simulink model "prob1"  (R2020b)
settings: Solver=VariableStepAuto  StartTime=0.0  StopTime=10.0  RelTol=1e-3
undefined symbols (not defined in the file): M1
settings Model: Creator=nadee  LastModifiedBy=nadee

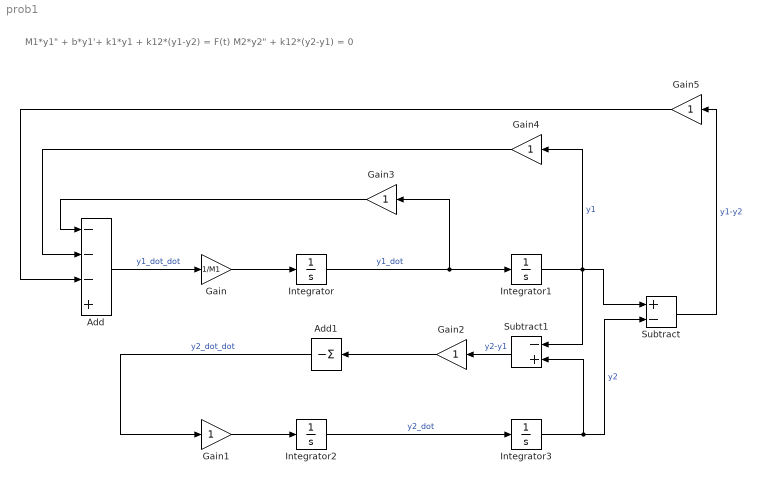
== system prob1 ==
  note: M1*y1" + b*y1'+ k1*y1 + k12*(y1-y2) = F(t)
      | M2*y2" + k12*(y2-y1) = 0
  Add : Sum  Inputs=---+
  Add1 : Sum  Inputs=-
  Gain : Gain  Gain=1/M1
  Gain{1..5} (5 alike) : Gain
  Integrator{,1..3} (4 alike) : Integrator
  Subtract : Sum  Inputs=+-
  Subtract1 : Sum  Inputs=-+
  wires:
  Integrator/1 -> Gain3/1, Integrator1/1  "y1_dot"
  Integrator1/1 -> Gain4/1, Subtract/1, Subtract1/1  "y1"
  Integrator3/1 -> Subtract1/2, Subtract/2  "y2"
  Integrator2/1 -> Integrator3/1  "y2_dot"
  Gain1/1 -> Integrator2/1
  Add1/1 -> Gain1/1  "y2_dot_dot"
  Gain2/1 -> Add1/1
  Subtract1/1 -> Gain2/1  "y2-y1"
  Gain/1 -> Integrator/1
  Add/1 -> Gain/1  "y1_dot_dot"
  Subtract/1 -> Gain5/1  "y1-y2"
  Gain5/1 -> Add/3
  Gain4/1 -> Add/2
  Gain3/1 -> Add/1
